simulink model "uchyby_sim"  (R2018a)
settings: Solver=VariableStepAuto  StartTime=0.0  StopTime=10.0  RelTol=1e-3
values from neighbouring files (symbols this model uses):
  k1 = -30    [uchyb.m]
  k2 = 30    [uchyb.m]
  k3 = 90    [uchyb.m]
settings Model: Creator=johnb  LastModifiedBy=johnb

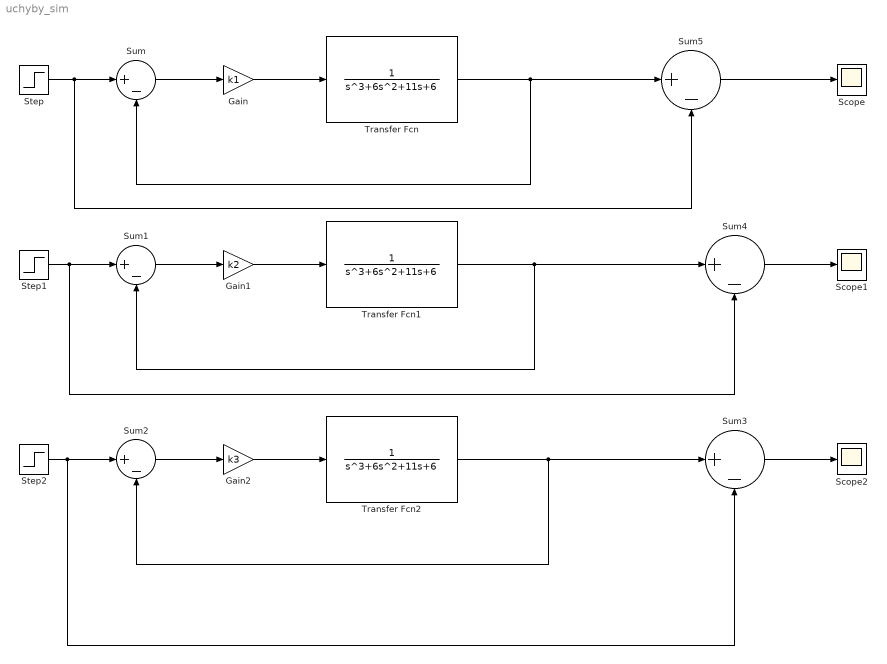
== system uchyby_sim ==
  Gain : Gain  Gain=k1
  Gain1 : Gain  Gain=k2
  Gain2 : Gain  Gain=k3
  Scope : Scope
  Scope1 : Scope
  Scope2 : Scope
  Step : Step  SampleTime=0
  Step1 : Step  SampleTime=0
  Step2 : Step  SampleTime=0
  Sum{,1..5} (6 alike) : Sum  Inputs=|+-
  Transfer Fcn : TransferFcn  Denominator=[1 6 11 6]
  Transfer Fcn1 : TransferFcn  Denominator=[1 6 11 6]
  Transfer Fcn2 : TransferFcn  Denominator=[1 6 11 6]
  wires:
  Transfer Fcn/1 -> Sum5/1, Sum/2
  Sum/1 -> Gain/1
  Gain/1 -> Transfer Fcn/1
  Sum1/1 -> Gain1/1
  Transfer Fcn1/1 -> Sum4/1, Sum1/2
  Gain1/1 -> Transfer Fcn1/1
  Sum2/1 -> Gain2/1
  Transfer Fcn2/1 -> Sum3/1, Sum2/2
  Gain2/1 -> Transfer Fcn2/1
  Step2/1 -> Sum3/2, Sum2/1
  Sum3/1 -> Scope2/1
  Step1/1 -> Sum4/2, Sum1/1
  Step/1 -> Sum5/2, Sum/1
  Sum5/1 -> Scope/1
  Sum4/1 -> Scope1/1
